simulink model "model_response"  (R2024b)
settings: Solver=VariableStepAuto  StartTime=0.0  StopTime=10.0  RelTol=1e-3
undefined symbols (not defined in the file): F, K, SS, u_amp, u_w, useSine
settings Model: Creator=carso  LastModifiedBy=carso

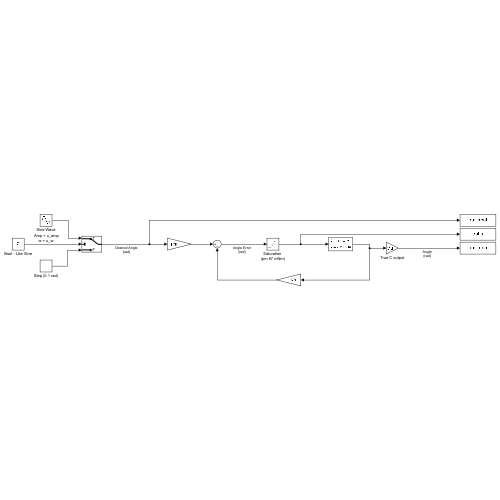
[thumbnail: Simulink's stored preview of the top-level diagram]
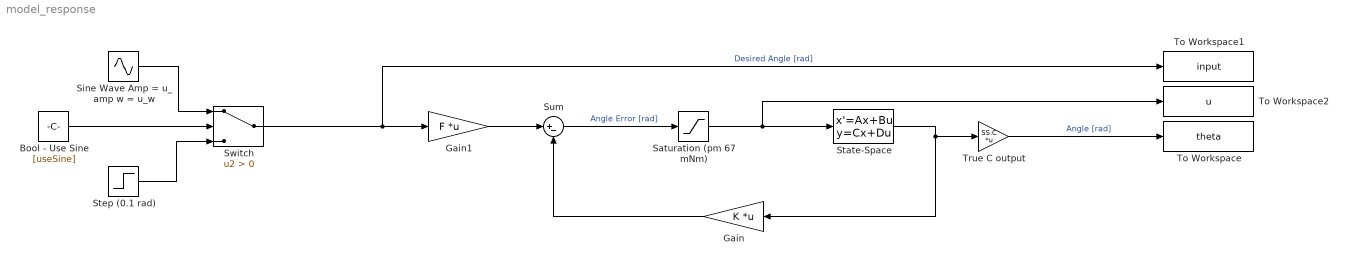
== system model_response ==
  Bool - Use Sine : Constant  Value=[useSine]
  Gain : Gain  Gain=K  Multiplication=Matrix(K*u)
  Gain1 : Gain  Gain=F  Multiplication=Matrix(K*u)
  Saturation (pm 67 mNm) : Saturate  UpperLimit=67  LowerLimit=-67
  Sine Wave Amp = u_amp w = u_w : Sin  Amplitude=[u_amp]  Frequency=[u_w]  SampleTime=0
  State-Space : StateSpace  A=SS.A  B=SS.B  C=eye(4)  D=zeros(4,1)  InitialCondition=0
  Step (0.1 rad) : Step  After=0.1  SampleTime=0
  Sum : Sum  Inputs=|+-
  Switch : Switch  Criteria=u2 > Threshold  SaturateOnIntegerOverflow=off  InputSameDT=off
  To Workspace : ToWorkspace  VariableName=theta  SaveFormat=Timeseries  SampleTime=-1
  To Workspace1 : ToWorkspace  VariableName=input  SaveFormat=Timeseries  SampleTime=-1
  To Workspace2 : ToWorkspace  VariableName=u  SaveFormat=Timeseries  SampleTime=-1
  True C output : Gain  Gain=SS.C  Multiplication=Matrix(K*u)
  wires:
  Sum/1 -> Saturation (pm 67 mNm)/1  "Angle Error [rad]"
  True C output/1 -> To Workspace/1  "Angle [rad]"
  Switch/1 -> To Workspace1/1, Gain1/1  "Desired Angle [rad]"
  Bool - Use Sine/1 -> Switch/2
  Step (0.1 rad)/1 -> Switch/3
  Sine Wave Amp = u_amp w = u_w/1 -> Switch/1
  Saturation (pm 67 mNm)/1 -> To Workspace2/1, State-Space/1
  Gain/1 -> Sum/2
  State-Space/1 -> True C output/1, Gain/1
  Gain1/1 -> Sum/1
